simulink library "csbenchlab_est"  (R2024a)
settings: Solver=VariableStepAuto  StartTime=0.0  StopTime=10.0  RelTol=1e-3
undefined symbols (not defined in the file or in its folder): extrinsic, PropagateState_data, PropagateState_DT, PropagateState_params, PropagateState_PT
settings Model: Creator=luka  LastModifiedBy=luka

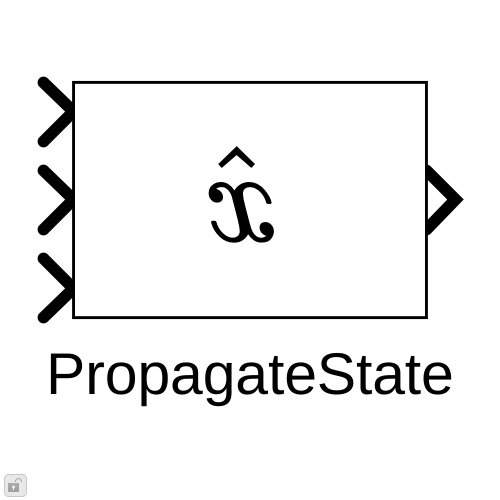
[thumbnail: Simulink's stored preview of the top-level diagram]
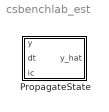
== system csbenchlab_est ==
  PropagateState : Subsystem  Tag=__cs_m_est;  mask{params=PropagateState_params, data=PropagateState_data, ParamsType=PropagateState_PT, DataType=PropagateState_DT, iid__=[0], pid__=[80 114 111 112 97 103 97 116 101 83 116 97 116 101 58 99 115 98 101 110 99 104 108 97 98]}
      mask prompts: params "Parameter struct:"

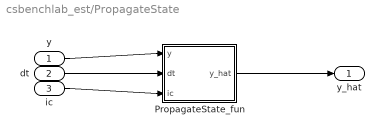
== system csbenchlab_est/PropagateState ==
  y : Inport
  dt : Inport  Port=2
  ic : Inport  Port=3
  PropagateState_fun : MATLAB Function  TreatAsAtomicUnit=on
  y_hat : Outport
  wires:
  y/1 -> PropagateState_fun/1(y)
  dt/1 -> PropagateState_fun/2(dt)
  ic/1 -> PropagateState_fun/3(ic)
  PropagateState_fun/1(y_hat) -> y_hat/1

== matlab function csbenchlab_est/PropagateState/PropagateState_fun ==
  settings: updateMethod=DISCRETE
  data: y input; y_hat output; dt input; ic input; extrinsic parameter int32; iid__ parameter uint8; pid__ parameter uint8; data parameter DataType; params parameter ParamsType
% __classname:="PropagateState";
% __fnname:="fcn_eaf8903c39704b0aa4a16e21ac53578c";
% __input_args:="y, dt, ic, params, data, pid__, iid__";
% __output_args:=" y_hat";
% __ctor_args:="params, 'Data', data, 'pid', pid__, 'iid', iid__";
% __cfg_args:=" ic";
% __step_args:="y, dt";
function y_hat = fcn(y, dt, ic, extrinsic, iid__, pid__, data, params)
  coder.extrinsic('fcn_eaf8903c39704b0aa4a16e21ac53578c_ext');
  if extrinsic
      y_hat = zeros(size(ic));
      y_hat = fcn_eaf8903c39704b0aa4a16e21ac53578c_ext(y, dt, ic, params, data, pid__, iid__);
  else
      y_hat = fcn_eaf8903c39704b0aa4a16e21ac53578c(y, dt, ic, params, data, pid__, iid__);
  end
end

function y_hat = fcn_eaf8903c39704b0aa4a16e21ac53578c(y, dt, ic, params, data, pid__, iid__)
  persistent obj
  if isempty(obj)
    obj = PropagateState(params, 'Data', data, 'pid', pid__, 'iid', iid__);
    obj = obj.configure( ic);
  end
  [obj, y_hat] = obj.step(y, dt);
end
